simulink model "mrsMecanumModel"  (R2018a)
settings: Solver=VariableStepAuto  StartTime=0.0  StopTime=inf  FixedStep=0.01  RelTol=1e-3  EnableMultiTasking=on
PreLoadFcn:
  | sampleTime = 0.05;
  | 
  | % Vehicle Parameters
  | wheelRadius = 0.1;
  | wheelBase = 0.4;
  | wheelTrack = 0.5;
libraries: mobileRoboticsLib x4
settings Model: EnablePacing=on  Creator=scastro  LastModifiedBy=scastro
settings DataIOCC: LimitDataPoints=on
settings OptimizationCC: LifeSpan=inf
settings DebuggingCC: AllowSymbolicDim=off  SFUnexpectedBacktrackingDiag=warning  SFNoUnconditionalDefaultTransitionDiag=warning  SFExecutionAtInitializationDiag=none
settings CodeAppCC: StateflowObjectComments=on
settings GRTTargetCC: TargetLangStandard=C89/C90 (ANSI)  GeneratePreprocessorConditionals=Disable all
settings ConfigComp: CovMetricSettings=dw  CovHtmlReporting=on  CovSaveCumulativeToWorkspaceVar=on  CovSaveSingleToWorkspaceVar=on  CovExternalEMLEnable=off  CovSFcnEnable=off
settings SimscapeCC: SimscapeNominalValues="[{\"value\":\"10\",\"unit\":\"V\"},{\"value\":\"1\",\"unit\":\"A\"},{\"value\":\"10\",\"unit\":\"N*m\"},{\"value\":\"10\",\"unit\":\"bar\"},{\"value\":\"100\",\"unit\":\"kJ/kg\"},{\"value\":\"1\",\"unit\":\"kW\"},{\"value\":\"300\",\"unit\":\"K\"},{\"value\":\"100\",\"unit\":\"cm^3/s\"},{\"value\":\"1\",\"unit\":\"kN\"},{\"value\":\"1\",\"unit\":\"g/cm^3\"},{\"value\":\"1\",\"unit\":\"l\"},{\"value\":\"1\",\"unit\":\"cm^2\"},{\"value\":\"60\",\"unit\":\"Hz\"}]"  SimscapeLogType=all  SimscapeLogDataHistory=10000
settings ConfigurationSet: Description=SimMechanics 2G
settings ExplorerConfigSet: InternalSimMechanicsExplorerSettings="<ExplorerConfiguration><canonicalview>default</canonicalview><AnimationSetting><BasePlaybackSpeed>1.0</BasePlaybackSpeed><PlaybackSpeedFactor>1.0</PlaybackSpeedFactor></AnimationSetting><TilePanel><TileInfo><Tiles Columns=\"1\" Count=\"1\" Rows=\"1\"><Column Weight=\"1\"/><Row Weight=\"1\"/><Tile Height=\"1\" Width=\"1\" X=\"0\" Y=\"0\"/></Tiles></TileInfo><SceneInfo><SceneViewer><BGColor><R>0.60000002384185791</R><G>0.60000002384185791</G><B>0.60000002384185791</B></BGColor><Camera><DoPerspective>off</DoPerspective><Position><X>-1.70656042355848525</X><Y>-0.974920623359631922</Y><Z>4.72930454537082046</Z></Position><Center><X>0.552860638431633689</X><Y>1.42025063411503494</Y><Z>1.4843509506914252</Z></Center><Up><X>0.664249622453917166</X><Y>0.300615402055903091</Y><Z>0.684399604848363485</Z></Up><ViewLimDist>1</ViewLimDist><YLim>2.77881717169207398</YLim><XLim>3.55928742670435394</XLim></Camera></SceneViewer></SceneInfo></TilePanel><MechEditorPanel><Cameras/><GfxPanelCameraMap/><VideoCreator><PlaybackSpeedRatio>1.0</PlaybackSpeedRatio><FrameRate>30</FrameRate><VideoFormat>Motion JPEG AVI</VideoFormat><FrameSize>auto</FrameSize></VideoCreator></MechEditorPanel></ExplorerConfiguration>"

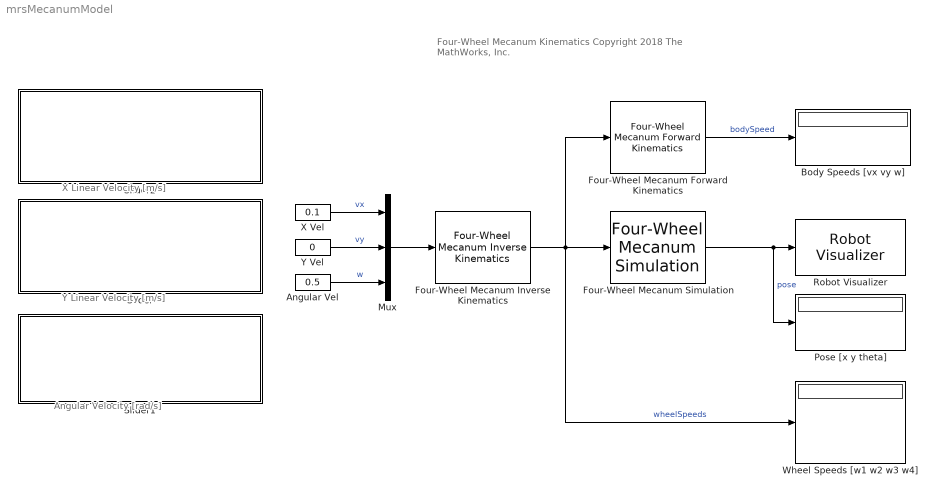
== system mrsMecanumModel ==
  note: Y Linear Velocity [m/s]
  note: Angular Velocity [rad/s]
  note: X Linear Velocity [m/s]
  note: Four-Wheel Mecanum Kinematics
      |
      | Copyright 2018 The MathWorks, Inc.
  Angular Vel : Constant  Value=0.5
  Body Speeds [vx vy w] : Display
  Four-Wheel Mecanum Forward Kinematics : mobileRoboticsLib/Kinematic Models/Four-Wheel Mecanum/Four-Wheel Mecanum Forward Kinematics  wheelRadius=wheelRadius  wheelBase=wheelBase  wheelTrack=wheelTrack
      settings: SourceProductName=Mobile Robotics Simulation Library
  Four-Wheel Mecanum Inverse Kinematics : mobileRoboticsLib/Kinematic Models/Four-Wheel Mecanum/Four-Wheel Mecanum Inverse Kinematics  wheelRadius=wheelRadius  wheelBase=wheelBase  wheelTrack=wheelTrack
      settings: SourceProductName=Mobile Robotics Simulation Library
  Four-Wheel Mecanum Simulation : mobileRoboticsLib/Kinematic Models/Four-Wheel Mecanum/Four-Wheel Mecanum Simulation  OverrideUsingVariant=mode==2  wheelRadius=wheelRadius  wheelBase=wheelBase  wheelTrack=wheelTrack  initX=0  initY=0  initAngle=0  Ts=sampleTime
      settings: SourceProductName=Mobile Robotics Simulation Library
  Mux : Mux  Inputs=3
  Pose [x y theta] : Display
  Robot Visualizer : mobileRoboticsLib/Environments/Robot Visualizer  Priority=99  showTrajectory=on  hasWaypoints=off  hasLidar=off  sensorOffset=[ 0 0 ]  scanAngles=scanAngles  hasObjDetector=off  objDetectorOffset=[ 0, 0 ]  objDetectorAngle=0  objDetectorFOV=pi/4  objDetectorMaxRange=5  objectColors=[ 1, 0, 0; 0, 1, 0; 0, 0, 1 ]
      settings: SourceProductName=Ground Vehicles Library
  Slider : Subsystem  DialogController=hmiCreateDDGDialog  IsWebBlock=on  mask(MWDashboardBlock){webBlockId=91029beb-32c8-459e-a49c-538ef9bb95ac, webBlockType=slider, ShowInLibBrowser=on, ShowInitialText=on, HMISrcModelName=mrsMecanumModel}
      mask prompts: webBlockId "WebBlock Id"; webBlockType "WebBlock Type"; HMISrcModelName "Source Model"
      mask help: SimulinkHMI:dialogs:SliderDialogDesc
      mask Help: helpview([docroot '/mapfiles/simulink.map'], 'hmi_slider')
      mask Display:
      | if strcmp(get_param(bdroot(gcb),'BlockDiagramType'), 'library')
      |     image([(matlabroot) '/toolbox/simulink/hmi/icons/Slider.png']);
      | end
  Slider1 : Subsystem  DialogController=hmiCreateDDGDialog  IsWebBlock=on  mask(MWDashboardBlock){webBlockId=57621d3f-6b07-4592-bbca-6acf347e8acf, webBlockType=slider, ShowInLibBrowser=on, ShowInitialText=on, HMISrcModelName=mrsMecanumModel}
      mask prompts: webBlockId "WebBlock Id"; webBlockType "WebBlock Type"; HMISrcModelName "Source Model"
      mask help: SimulinkHMI:dialogs:SliderDialogDesc
      mask Help: helpview([docroot '/mapfiles/simulink.map'], 'hmi_slider')
      mask Display:
      | if strcmp(get_param(bdroot(gcb),'BlockDiagramType'), 'library')
      |     image([(matlabroot) '/toolbox/simulink/hmi/icons/Slider.png']);
      | end
  Slider2 : Subsystem  DialogController=hmiCreateDDGDialog  IsWebBlock=on  mask(MWDashboardBlock){webBlockId=a161dc59-9716-4089-a7a1-689fff0a577a, webBlockType=slider, ShowInLibBrowser=on, ShowInitialText=on, HMISrcModelName=mrsMecanumModel}
      mask prompts: webBlockId "WebBlock Id"; webBlockType "WebBlock Type"; HMISrcModelName "Source Model"
      mask help: SimulinkHMI:dialogs:SliderDialogDesc
      mask Help: helpview([docroot '/mapfiles/simulink.map'], 'hmi_slider')
      mask Display:
      | if strcmp(get_param(bdroot(gcb),'BlockDiagramType'), 'library')
      |     image([(matlabroot) '/toolbox/simulink/hmi/icons/Slider.png']);
      | end
  Wheel Speeds [w1 w2 w3 w4] : Display
  X Vel : Constant  Value=0.1
  Y Vel : Constant  Value=0
  wires:
  Four-Wheel Mecanum Inverse Kinematics/1 -> Four-Wheel Mecanum Forward Kinematics/1, Four-Wheel Mecanum Simulation/1, Wheel Speeds [w1 w2 w3 w4]/1  "wheelSpeeds"
  Angular Vel/1 -> Mux/3  "w"
  Mux/1 -> Four-Wheel Mecanum Inverse Kinematics/1
  X Vel/1 -> Mux/1  "vx"
  Four-Wheel Mecanum Simulation/1 -> Pose [x y theta]/1, Robot Visualizer/1  "pose"
  Y Vel/1 -> Mux/2  "vy"
  Four-Wheel Mecanum Forward Kinematics/1 -> Body Speeds [vx vy w]/1  "bodySpeed"

== system mrsMecanumModel/Slider ==

== system mrsMecanumModel/Slider1 ==

== system mrsMecanumModel/Slider2 ==
